simulink library "Logic_Operations_Lib"  (Simulink 8.1)
settings: Solver=ode45  StartTime=0.0  StopTime=10.0  RelTol=1e-3
libraries: commutil2 x11
settings Model: Creator=uzivatel  LastModifiedBy=uzivatel

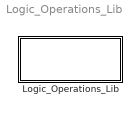
== system Logic_Operations_Lib ==
  Logic_Operations_Lib : Subsystem

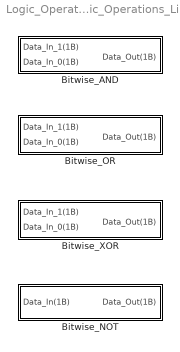
== system Logic_Operations_Lib/Logic_Operations_Lib ==
  Bitwise_AND : Subsystem
  Bitwise_NOT : Subsystem
  Bitwise_OR : Subsystem
  Bitwise_XOR : Subsystem

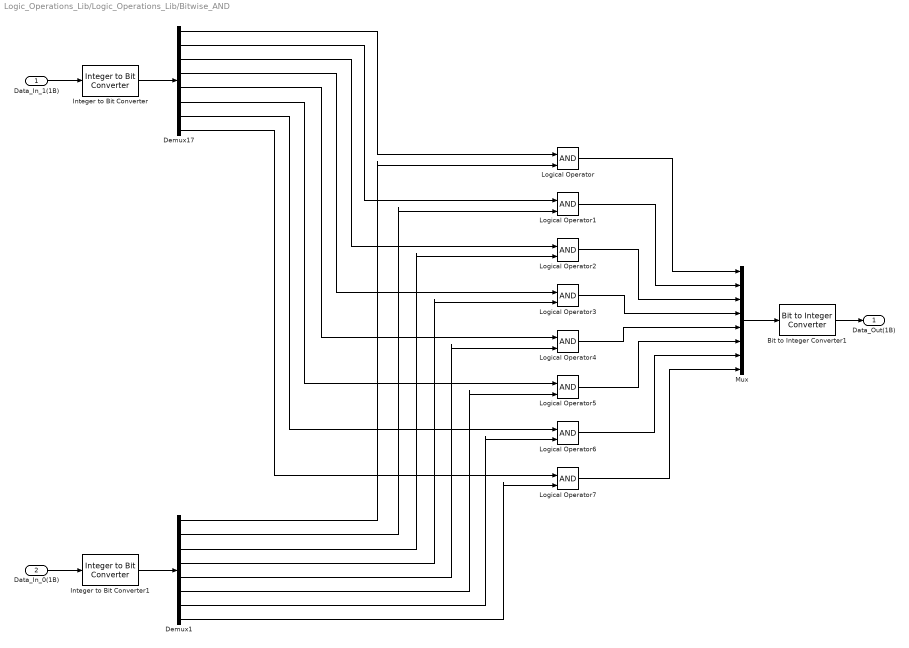
== system Logic_Operations_Lib/Logic_Operations_Lib/Bitwise_AND ==
  Data_In_1(1B) : Inport
  Data_In_0(1B) : Inport  Port=2
  Bit to Integer Converter1 : commutil2/Bit to Integer Converter  nbits=8  bitOrder=MSB first  signedOutputValues=Unsigned  outDtype=uint8  outDtypeSigned=Inherit via internal rule
  Demux1 : Demux  Outputs=8
  Demux17 : Demux  Outputs=8
  Integer to Bit Converter : commutil2/Integer to Bit Converter  nbits=8  signedInputValues=Unsigned  bitOrder=MSB first  outDtype=boolean
  Integer to Bit Converter1 : commutil2/Integer to Bit Converter  nbits=8  signedInputValues=Unsigned  bitOrder=MSB first  outDtype=boolean
  Logical Operator{,1..7} (8 alike) : Logic  IconShape=distinctive  AllPortsSameDT=off  OutDataTypeStr=boolean
  Mux : Mux  Inputs=8
  Data_Out(1B) : Outport
  wires:
  Data_In_1(1B)/1 -> Integer to Bit Converter/1
  Data_In_0(1B)/1 -> Integer to Bit Converter1/1
  Demux17/1 -> Logical Operator/1
  Demux1/1 -> Logical Operator/2
  Demux17/2 -> Logical Operator1/1
  Demux1/2 -> Logical Operator1/2
  Demux1/3 -> Logical Operator2/2
  Demux17/3 -> Logical Operator2/1
  Demux17/4 -> Logical Operator3/1
  Demux1/4 -> Logical Operator3/2
  Demux17/5 -> Logical Operator4/1
  Demux1/5 -> Logical Operator4/2
  Demux17/6 -> Logical Operator5/1
  Demux1/6 -> Logical Operator5/2
  Demux17/7 -> Logical Operator6/1
  Demux1/7 -> Logical Operator6/2
  Demux17/8 -> Logical Operator7/1
  Demux1/8 -> Logical Operator7/2
  Mux/1 -> Bit to Integer Converter1/1
  Logical Operator4/1 -> Mux/5
  Logical Operator3/1 -> Mux/4
  Logical Operator5/1 -> Mux/6
  Logical Operator6/1 -> Mux/7
  Logical Operator7/1 -> Mux/8
  Logical Operator2/1 -> Mux/3
  Logical Operator1/1 -> Mux/2
  Logical Operator/1 -> Mux/1
  Integer to Bit Converter/1 -> Demux17/1
  Integer to Bit Converter1/1 -> Demux1/1
  Bit to Integer Converter1/1 -> Data_Out(1B)/1

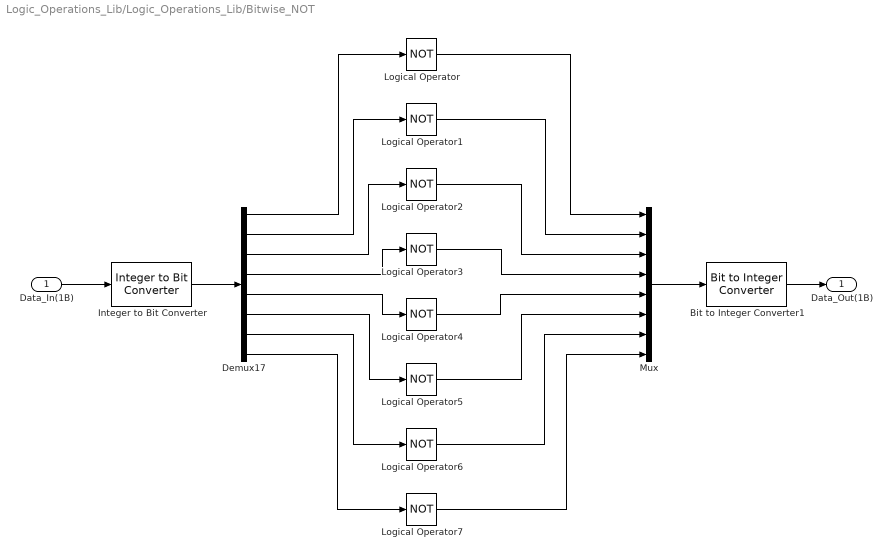
== system Logic_Operations_Lib/Logic_Operations_Lib/Bitwise_NOT ==
  Data_In(1B) : Inport
  Bit to Integer Converter1 : commutil2/Bit to Integer Converter  nbits=8  bitOrder=MSB first  signedOutputValues=Unsigned  outDtype=uint8  outDtypeSigned=Inherit via internal rule
  Demux17 : Demux  Outputs=8
  Integer to Bit Converter : commutil2/Integer to Bit Converter  nbits=8  signedInputValues=Unsigned  bitOrder=MSB first  outDtype=boolean
  Logical Operator{,1..7} (8 alike) : Logic  Operator=NOT  IconShape=distinctive  AllPortsSameDT=off  OutDataTypeStr=boolean
  Mux : Mux  Inputs=8
  Data_Out(1B) : Outport
  wires:
  Integer to Bit Converter/1 -> Demux17/1
  Demux17/1 -> Logical Operator/1
  Demux17/2 -> Logical Operator1/1
  Demux17/3 -> Logical Operator2/1
  Demux17/4 -> Logical Operator3/1
  Demux17/5 -> Logical Operator4/1
  Demux17/6 -> Logical Operator5/1
  Demux17/7 -> Logical Operator6/1
  Demux17/8 -> Logical Operator7/1
  Mux/1 -> Bit to Integer Converter1/1
  Logical Operator4/1 -> Mux/5
  Logical Operator3/1 -> Mux/4
  Logical Operator5/1 -> Mux/6
  Logical Operator6/1 -> Mux/7
  Logical Operator7/1 -> Mux/8
  Logical Operator2/1 -> Mux/3
  Logical Operator1/1 -> Mux/2
  Logical Operator/1 -> Mux/1
  Data_In(1B)/1 -> Integer to Bit Converter/1
  Bit to Integer Converter1/1 -> Data_Out(1B)/1

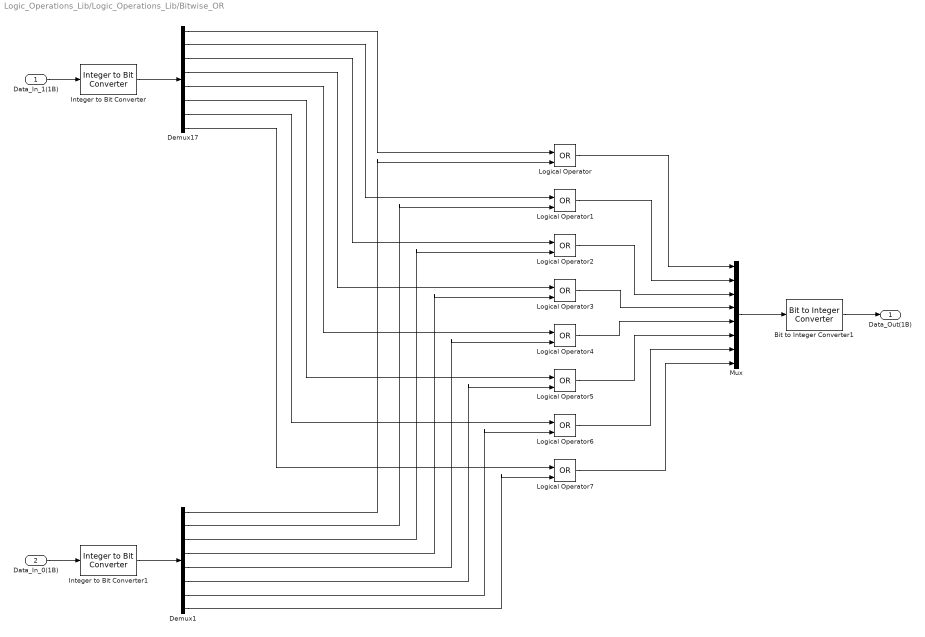
== system Logic_Operations_Lib/Logic_Operations_Lib/Bitwise_OR ==
  Data_In_1(1B) : Inport
  Data_In_0(1B) : Inport  Port=2
  Bit to Integer Converter1 : commutil2/Bit to Integer Converter  nbits=8  bitOrder=MSB first  signedOutputValues=Unsigned  outDtype=uint8  outDtypeSigned=Inherit via internal rule
  Demux1 : Demux  Outputs=8
  Demux17 : Demux  Outputs=8
  Integer to Bit Converter : commutil2/Integer to Bit Converter  nbits=8  signedInputValues=Unsigned  bitOrder=MSB first  outDtype=boolean
  Integer to Bit Converter1 : commutil2/Integer to Bit Converter  nbits=8  signedInputValues=Unsigned  bitOrder=MSB first  outDtype=boolean
  Logical Operator{,1..7} (8 alike) : Logic  Operator=OR  IconShape=distinctive  AllPortsSameDT=off  OutDataTypeStr=boolean
  Mux : Mux  Inputs=8
  Data_Out(1B) : Outport
  wires:
  Integer to Bit Converter/1 -> Demux17/1
  Integer to Bit Converter1/1 -> Demux1/1
  Demux17/1 -> Logical Operator/1
  Demux1/1 -> Logical Operator/2
  Demux17/2 -> Logical Operator1/1
  Demux1/2 -> Logical Operator1/2
  Demux1/3 -> Logical Operator2/2
  Demux17/3 -> Logical Operator2/1
  Demux17/4 -> Logical Operator3/1
  Demux1/4 -> Logical Operator3/2
  Demux17/5 -> Logical Operator4/1
  Demux1/5 -> Logical Operator4/2
  Demux17/6 -> Logical Operator5/1
  Demux1/6 -> Logical Operator5/2
  Demux17/7 -> Logical Operator6/1
  Demux1/7 -> Logical Operator6/2
  Demux17/8 -> Logical Operator7/1
  Demux1/8 -> Logical Operator7/2
  Logical Operator4/1 -> Mux/5
  Logical Operator3/1 -> Mux/4
  Logical Operator5/1 -> Mux/6
  Logical Operator6/1 -> Mux/7
  Logical Operator7/1 -> Mux/8
  Logical Operator2/1 -> Mux/3
  Logical Operator1/1 -> Mux/2
  Logical Operator/1 -> Mux/1
  Data_In_1(1B)/1 -> Integer to Bit Converter/1
  Data_In_0(1B)/1 -> Integer to Bit Converter1/1
  Bit to Integer Converter1/1 -> Data_Out(1B)/1
  Mux/1 -> Bit to Integer Converter1/1

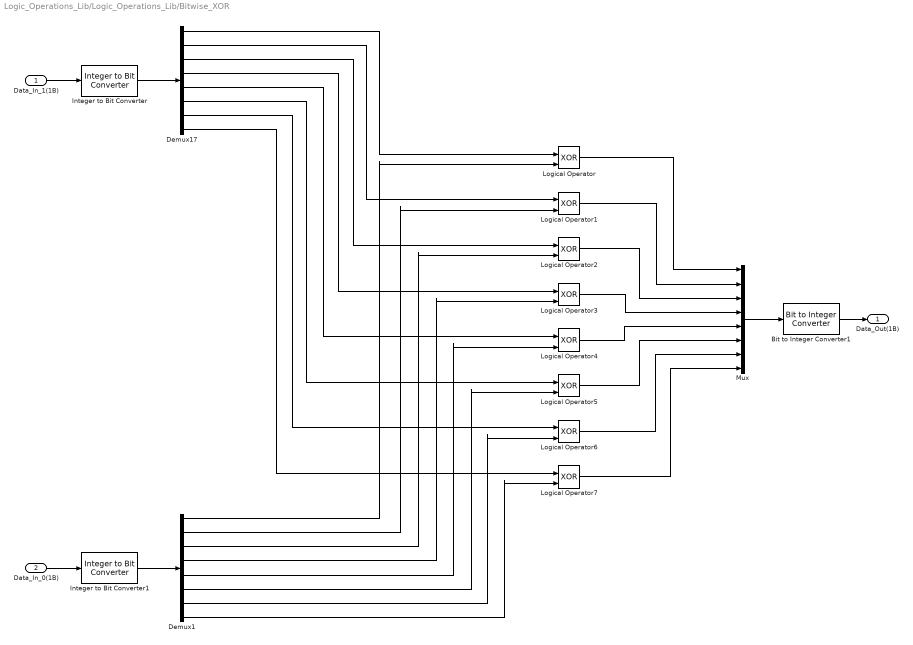
== system Logic_Operations_Lib/Logic_Operations_Lib/Bitwise_XOR ==
  Data_In_1(1B) : Inport
  Data_In_0(1B) : Inport  Port=2
  Bit to Integer Converter1 : commutil2/Bit to Integer Converter  nbits=8  bitOrder=MSB first  signedOutputValues=Unsigned  outDtype=uint8  outDtypeSigned=Inherit via internal rule
  Demux1 : Demux  Outputs=8
  Demux17 : Demux  Outputs=8
  Integer to Bit Converter : commutil2/Integer to Bit Converter  nbits=8  signedInputValues=Unsigned  bitOrder=MSB first  outDtype=boolean
  Integer to Bit Converter1 : commutil2/Integer to Bit Converter  nbits=8  signedInputValues=Unsigned  bitOrder=MSB first  outDtype=boolean
  Logical Operator{,1..7} (8 alike) : Logic  Operator=XOR  IconShape=distinctive  AllPortsSameDT=off  OutDataTypeStr=boolean
  Mux : Mux  Inputs=8
  Data_Out(1B) : Outport
  wires:
  Integer to Bit Converter/1 -> Demux17/1
  Integer to Bit Converter1/1 -> Demux1/1
  Demux17/1 -> Logical Operator/1
  Demux1/1 -> Logical Operator/2
  Demux17/2 -> Logical Operator1/1
  Demux1/2 -> Logical Operator1/2
  Demux1/3 -> Logical Operator2/2
  Demux17/3 -> Logical Operator2/1
  Demux17/4 -> Logical Operator3/1
  Demux1/4 -> Logical Operator3/2
  Demux17/5 -> Logical Operator4/1
  Demux1/5 -> Logical Operator4/2
  Demux17/6 -> Logical Operator5/1
  Demux1/6 -> Logical Operator5/2
  Demux17/7 -> Logical Operator6/1
  Demux1/7 -> Logical Operator6/2
  Demux17/8 -> Logical Operator7/1
  Demux1/8 -> Logical Operator7/2
  Mux/1 -> Bit to Integer Converter1/1
  Logical Operator4/1 -> Mux/5
  Logical Operator3/1 -> Mux/4
  Logical Operator5/1 -> Mux/6
  Logical Operator6/1 -> Mux/7
  Logical Operator7/1 -> Mux/8
  Logical Operator2/1 -> Mux/3
  Logical Operator1/1 -> Mux/2
  Logical Operator/1 -> Mux/1
  Data_In_1(1B)/1 -> Integer to Bit Converter/1
  Data_In_0(1B)/1 -> Integer to Bit Converter1/1
  Bit to Integer Converter1/1 -> Data_Out(1B)/1
